simulink model "Project_PI_example_part3"  (R2020a)
settings: Solver=ode4  StartTime=0  StopTime=4.8  FixedStep=5e-6  MaxStep=1e-6  RelTol=1e-6  AbsTol=1e-6  EnableMultiTasking=on
PreLoadFcn:
  | assignin('base','Ts',[5e-6])
values from neighbouring files (symbols this model uses):
  integral_term = .025    (= 0.025)    [PI_contolled_pwm_part3.m]    (also in PI_controlled_pwm.m; PI_controlled_sinpwm.m; motor3.m = 1)
  proportional_term = 40    [PI_contolled_pwm_part3.m]    (also in PI_controlled_pwm.m; PI_controlled_sinpwm.m; motor3.m = 1)
libraries: powerlib x14, simulink x3
Description:
  | This example illustrates use of the BLDC in a closed-loop
  | speed and voltage control on a 1 kW, 3000 rpm industrial motor
  | 
  | 
  | Copyright 2008-2017 The MathWorks, Inc.
settings Model: ExtModeAutoUpdateStatusClock=off  Creator=MathWorks  LastModifiedBy=gapaul
settings SolverCC: AutoScaleAbsTol=off
settings DataIOCC: SaveFormat=Array  SignalLoggingSaveFormat=ModelDataLogs  ReturnWorkspaceOutputs=off  SignalLoggingName=sigsOut
settings OptimizationCC: ExpressionDepthLimit=2147483647  InitFltsAndDblsToZero=on  LifeSpan=inf
settings DebuggingCC: UnderspecifiedInitializationDetection=Classic  MergeDetectMultiDrivingBlocksExec=none  SignalResolutionControl=TryResolveAllWithWarning  MultiTaskDSMMsg=warning  MultiTaskCondExecSysMsg=none  FcnCallInpInsideContextMsg=warning  StateNameClashWarn=warning  SFUnexpectedBacktrackingDiag=warning  SFNoUnconditionalDefaultTransitionDiag=warning  SFExecutionAtInitializationDiag=none  ArithmeticOperatorsInVariantConditions=warning
settings HardwareCC: ProdBitPerPointer=32  ProdBitPerSizeT=32  ProdBitPerPtrDiffT=32  ProdLargestAtomicFloat=None  ProdIntDivRoundTo=Undefined  ProdEndianess=Unspecified  ProdWordSize=32  ProdHWDeviceType=32-bit Generic  TargetUnknown=on
settings ModelReferenceCC: PropagateSignalLabelsOutOfModel=off
settings SFSimCC: SimUseLocalCustomCode=off  CustomCodeUndefinedFunction=UseInterfaceOnly
settings RTWCC: RTWUseLocalCustomCode=off
settings CodeAppCC: StateflowObjectComments=on
settings GRTTargetCC: TargetLangStandard=C89/C90 (ANSI)  CombineOutputUpdateFcns=off  GRTInterface=on
settings ConfigComp: CovMetricSettings=dw  CovHtmlReporting=on  CovSaveCumulativeToWorkspaceVar=on  CovSaveSingleToWorkspaceVar=on  CovExternalEMLEnable=off  CovSFcnEnable=off
settings SimscapeCC: SimscapeNormalizeSystem=off

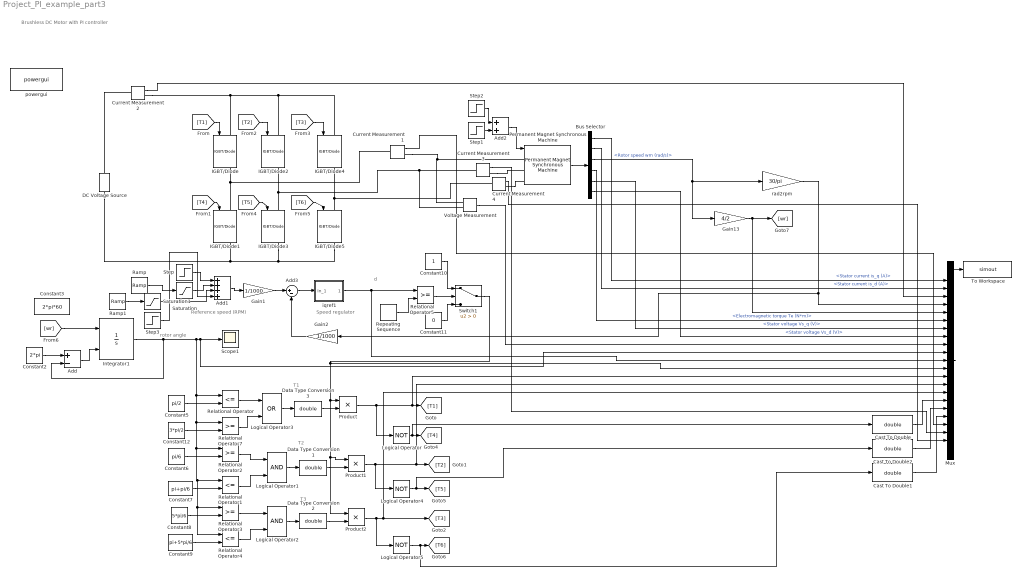
== system Project_PI_example_part3 ==
  note: d
  note: Brushless DC Motor with PI controller
  note: Speed
      | regulator
  note: Reference
      | speed (RPM)
  note: rotor angle
  note: T2
  note: T1
  note: T3
  Add : Sum  Inputs=+-
  Add1 : Sum  Inputs=++++
  Add2 : Sum
  Add3 : Sum  Inputs=|+-
  Bus Selector : BusSelector  OutputSignals=Stator current is_q (A),Stator current is_d (A),Rotor speed wm (rad/s),Electromagnetic torque Te (N*m),Stator voltage Vs_q (V),Stator voltage Vs_d (V)
  Cast To Double : DataTypeConversion  OutDataTypeStr=double
  Cast To Double1 : DataTypeConversion  OutDataTypeStr=double
  Cast To Double2 : DataTypeConversion  OutDataTypeStr=double
  Constant10 : Constant
  Constant11 : Constant  Value=0
  Constant12 : Constant  Value=3*pi/2
  Constant2 : Constant  Value=2*pi
  Constant3 : Constant  Value=2*pi*60
  Constant5 : Constant  Value=pi/2
  Constant6 : Constant  Value=pi/6
  Constant7 : Constant  Value=pi+pi/6
  Constant8 : Constant  Value=5*pi/6
  Constant9 : Constant  Value=pi+5*pi/6
  Current Measurement{1..4} (4 alike) : powerlib/Measurements/Current Measurement  PhasorSimulation=off  OutputType=Complex  PSBequivalent=0
  DC Voltage Source : powerlib/Electrical Sources/DC Voltage Source  Amplitude=72  Measurements=None
  Data Type Conversion1 : DataTypeConversion  OutDataTypeStr=double  SaturateOnIntegerOverflow=on  RndMeth=Zero
  Data Type Conversion2 : DataTypeConversion  OutDataTypeStr=double  SaturateOnIntegerOverflow=on  RndMeth=Zero
  Data Type Conversion3 : DataTypeConversion  OutDataTypeStr=double  SaturateOnIntegerOverflow=on  RndMeth=Zero
  Gain1 : Gain  Gain=1/1000
  Gain13 : Gain  Gain=4/2
  Gain2 : Gain  Gain=1/1000
  IGBT/Diode{,1..5} (6 alike) : powerlib/Power Electronics/IGBT//Diode  Ron=1e-5  Rs=1e5  Cs=inf  Measurements=on
  Integrator1 : Integrator  ExternalReset=falling
  Logical Operator : Logic  Operator=NOT  AllPortsSameDT=off  OutDataTypeStr=boolean
  Logical Operator1 : Logic  AllPortsSameDT=off  OutDataTypeStr=boolean
  Logical Operator2 : Logic  AllPortsSameDT=off  OutDataTypeStr=boolean
  Logical Operator3 : Logic  Operator=OR  AllPortsSameDT=off  OutDataTypeStr=boolean
  Logical Operator4 : Logic  Operator=NOT  AllPortsSameDT=off  OutDataTypeStr=boolean
  Logical Operator5 : Logic  Operator=NOT  AllPortsSameDT=off  OutDataTypeStr=boolean
  Mux : Mux  Inputs=21
  Permanent Magnet Synchronous Machine : powerlib/Machines/Permanent Magnet Synchronous Machine  NbPhases=3  FluxDistribution=Sinusoidal  RotorType=Round  MechanicalLoad=Torque Tm  PresetModel=No  ShowDetailedParameters=on  MeasurementBus=off  Resistance=3.4  Inductance=8.5e-3  dqInductances=[8.5e-3, 8.5e-3]  La=(1.1 + 3/2*11)*1e-3  MachineConstant=Flux linkage established by magnets (V.s)  Flux=0.2  VoltageCst=72.552  TorqueCst=0.6  Flat=120  Mechanical=[5e-4, 0 2]  PolePairs=4  InitialConditions=[0,0, 0,0]  InitialConditions5ph=[0 0 0 0 0 0]  RefAngle=90 degrees behind phase A axis (modified Park)  IterativeDiscreteModel=Trapezoidal non iterative  TsBlock=-1  TsPowergui=0
  Product : Product
  Product1 : Product
  Product2 : Product
  Ramp : simulink/Sources/Ramp  slope=500  start=0  InitialOutput=0
  Ramp1 : simulink/Sources/Ramp  slope=-500  start=2.8  InitialOutput=0
  Relational Operator : RelationalOperator  Operator=<=  OutDataTypeStr=boolean  RndMeth=Simplest
  Relational Operator1 : RelationalOperator  Operator=<=  OutDataTypeStr=boolean  RndMeth=Simplest
  Relational Operator{2..3,5,7} (4 alike) : RelationalOperator  OutDataTypeStr=boolean  RndMeth=Simplest
  Relational Operator4 : RelationalOperator  Operator=<=  OutDataTypeStr=boolean  RndMeth=Simplest
  Repeating Sequence : simulink/Sources/Repeating Sequence  rep_seq_t=[0 1e-3]  rep_seq_y=[0 1]
  Saturation : Saturate  UpperLimit=400  LowerLimit=0
  Saturation1 : Saturate  UpperLimit=0  LowerLimit=-461.5
  Scope1 : Scope
  Step : Step  Time=1.8  After=200  SampleTime=0
  Step1 : Step  Time=2.3  After=-2  SampleTime=0
  Step2 : Step  Time=1.3  Before=.5  SampleTime=0
  Step3 : Step  Time=4.223  After=-138.5  SampleTime=0
  Switch1 : Switch  Criteria=u2 > Threshold
  To Workspace : ToWorkspace  VariableName=simout  SaveFormat=Timeseries  SampleTime=-1
  Voltage Measurement : powerlib/Measurements/Voltage Measurement  PhasorSimulation=off  OutputType=Complex  PSBequivalent=0
  iqref1 : Subsystem  mask(PI Controller){I=integral_term, P=proportional_term, sat=[-10000, 10000]}
      mask prompts: I "Integral"; P "Proportional:"; sat "Minimum and maximum outputs:"
      mask init:
      | min=sat(1);max=sat(2);
      mask Display: disp('PI')
  powergui : powerlib/powergui  Priority=2  SimulationMode=Discrete  SampleTime=5e-6  frequency=60  Iterations=50  frequencyindice=0  Pbase=100e6  ErrMax=1e-4  UnitsV=kV  UnitsW=MW  buscounter=0  FunctionMessages=off  echomessages=off  EnableUseOfTLC=off  CurrentSourceSwitches=off  DisableSnubberDevices=off  DisableRonSwitches=off  DisableVfSwitches=off  DisplayEquations=off  AutomaticDiscreteSolvers=off  SolverType=Tustin/Backward Euler (TBE)  Interpol=off  ExternalGateDelay=off  methode=off  Ts=0  x0status=blocks  SPID=off  SwTol=0  HookPort=off  NonlinearTolerance=1e-4  nMaxIteration=100  ContinueOnMaxIteration=off  RestoreLinks=warning  ResistiveCurrentMeasurement=off  Frange=[0:2:500]  Ylog=off  Xlog=on  ShowGrid=off  save=off  variable=ZData  structure=0  ZoomFFT=on  StartTime=0.0  cycles=1  DisplayStyle=1  fundamental=60  FreqAxis=off  MaxFrequency=1000  frequencyindicesteady=1  RmsSteady=1  display=off
  rad2rpm : Gain  Gain=30/pi
  wires:
  Voltage Measurement/1 -> Mux/9
  Permanent Magnet Synchronous Machine/1 -> Bus Selector/1
  Bus Selector/3 -> Gain13/1, rad2rpm/1  "<Rotor speed wm (rad/s)>"
  [T4] -> IGBT/Diode1/1
  [T5] -> IGBT/Diode3/1
  [T6] -> IGBT/Diode5/1
  [T1] -> IGBT/Diode/1
  [T2] -> IGBT/Diode2/1
  [T3] -> IGBT/Diode4/1
  Constant2/1 -> Add/1
  Add/1 -> Integrator1/2
  [wr] -> Integrator1/1
  Relational Operator4/1 -> Logical Operator2/2
  Logical Operator2/1 -> Data Type Conversion2/1
  Relational Operator/1 -> Logical Operator3/1
  Relational Operator7/1 -> Logical Operator3/2
  Constant8/1 -> Relational Operator3/2
  Logical Operator1/1 -> Data Type Conversion1/1
  Relational Operator2/1 -> Logical Operator1/1
  Relational Operator1/1 -> Logical Operator1/2
  Logical Operator3/1 -> Data Type Conversion3/1
  Constant12/1 -> Relational Operator7/2
  Constant7/1 -> Relational Operator1/2
  Constant5/1 -> Relational Operator/2
  Integrator1/1 -> Mux/10, Scope1/1, Relational Operator/1, Relational Operator4/1, Relational Operator3/1, Relational Operator1/1, Relational Operator2/1, Relational Operator7/1, Add/2
  Relational Operator3/1 -> Logical Operator2/1
  Constant9/1 -> Relational Operator4/2
  Constant6/1 -> Relational Operator2/2
  Repeating Sequence/1 -> Relational Operator5/2
  Relational Operator5/1 -> Switch1/2
  Constant10/1 -> Switch1/1
  Constant11/1 -> Switch1/3
  Data Type Conversion3/1 -> Product/2
  Product/1 -> Logical Operator/1, Mux/13, [T1]
  Data Type Conversion1/1 -> Product1/2
  Product1/1 -> Mux/14, [T2], Logical Operator4/1
  Data Type Conversion2/1 -> Product2/2
  Product2/1 -> Logical Operator5/1, Mux/15, [T3]
  iqref1/1(Out_1) -> Mux/11, Relational Operator5/1
  Bus Selector/5 -> Mux/7  "<Stator voltage Vs_q (V)>"
  Bus Selector/6 -> Mux/8  "<Stator voltage Vs_d (V)>"
  Saturation/1 -> Add1/2
  Switch1/1 -> Product1/1, Product2/1, Product/1, Mux/12
  Gain1/1 -> Add3/1
  Gain2/1 -> Add3/2
  Current Measurement1/1 -> Mux/19
  Bus Selector/2 -> Mux/2  "<Stator current is_d (A)>"
  Cast To Double/1 -> Mux/16
  Cast To Double1/1 -> Mux/18
  Cast To Double2/1 -> Mux/17
  rad2rpm/1 -> Mux/4, Gain2/1
  Logical Operator4/1 -> Cast To Double2/1, [T5]
  Bus Selector/4 -> Mux/6  "<Electromagnetic torque Te (N*m)>"
  Logical Operator5/1 -> Cast To Double1/1, [T6]
  Gain13/1 -> Mux/5, [wr]
  Current Measurement2/1 -> Mux/3
  Mux/1 -> To Workspace/1
  Logical Operator/1 -> Cast To Double/1, [T4]
  Bus Selector/1 -> Mux/1  "<Stator current is_q (A)>"
  Add3/1 -> iqref1/1(In_1)
  Current Measurement3/1 -> Mux/20
  Current Measurement4/1 -> Mux/21
  Ramp/1 -> Saturation/1
  Add1/1 -> Gain1/1
  Step/1 -> Add1/1
  Ramp1/1 -> Saturation1/1
  Saturation1/1 -> Add1/3
  Step3/1 -> Add1/4
  Step1/1 -> Add2/2
  Step2/1 -> Add2/1
  Add2/1 -> Permanent Magnet Synchronous Machine/1
  connections:
  IGBT/Diode1/LConn1 -- Current Measurement1/LConn1 -- IGBT/Diode/RConn1
  IGBT/Diode2/RConn1 -- Current Measurement3/LConn1 -- Voltage Measurement/LConn2 -- IGBT/Diode3/LConn1
  IGBT/Diode4/RConn1 -- Current Measurement4/LConn1 -- IGBT/Diode5/LConn1
  IGBT/Diode1/RConn1 -- DC Voltage Source/LConn1 -- IGBT/Diode5/RConn1 -- IGBT/Diode3/RConn1
  IGBT/Diode2/LConn1 -- IGBT/Diode4/LConn1 -- IGBT/Diode/LConn1 -- Current Measurement2/RConn1
  Current Measurement2/LConn1 -- DC Voltage Source/RConn1
  Permanent Magnet Synchronous Machine/LConn1 -- Current Measurement1/RConn1 -- Voltage Measurement/LConn1
  Current Measurement3/RConn1 -- Permanent Magnet Synchronous Machine/LConn2
  Current Measurement4/RConn1 -- Permanent Magnet Synchronous Machine/LConn3

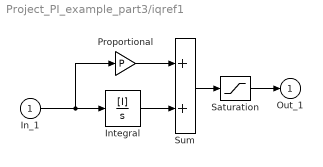
== system Project_PI_example_part3/iqref1 ==
  In_1 : Inport
  Integral : TransferFcn  Numerator=[I]  Denominator=[1 0]
  Proportional : Gain  Gain=P  SaturateOnIntegerOverflow=on  OutDataTypeStr=Inherit: Same as input  ParamDataTypeStr=Inherit: Same as input
  Saturation : Saturate  UpperLimit=max  LowerLimit=min
  Sum : Sum  InputSameDT=on  SaturateOnIntegerOverflow=on  OutDataTypeStr=Inherit: Same as first input
  Out_1 : Outport  InitialOutput=0  VectorParamsAs1DForOutWhenUnconnected=off
  wires:
  Saturation/1 -> Out_1/1
  Sum/1 -> Saturation/1
  Proportional/1 -> Sum/1
  In_1/1 -> Proportional/1, Integral/1
  Integral/1 -> Sum/2
